simulink library "mbed_targets_stm_arch_max"  (R2015a)
settings: Solver=ode45  StartTime=0.0  StopTime=10.0  RelTol=1e-3
libraries: mbed_lib x5, mbed_targets_stm_disco_f407 x1
settings Model: CovSFcnEnable=off  Creator=oh  LastModifiedBy=Stuv
settings DebuggingCC: SolverPrmCheckMsg=warning

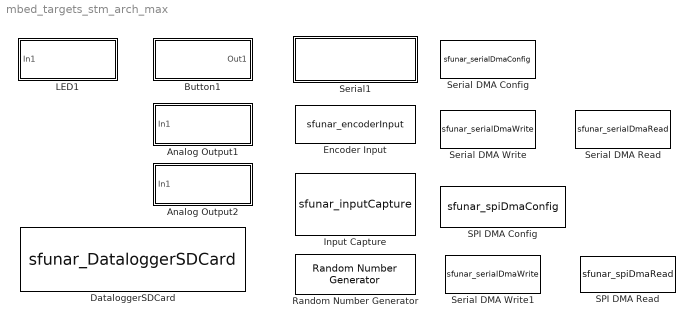
== system mbed_targets_stm_arch_max ==
  Analog Output1 : Subsystem  mask{Parameter1=0}
      mask Display:
      | offset=0.7;
      | plot([0+offset:0.025:0.25+offset],0.3*sin(2*pi*[0:0.1:1])+0.5)
      | port_label('input',1,['DAC1 (PA.4)']);
  Analog Output2 : Subsystem
      mask Display:
      | offset=0.7;
      | plot([0+offset:0.025:0.25+offset],0.3*sin(2*pi*[0:0.1:1])+0.5)
      | port_label('input',1,['DAC2 (PA.5)']);
  Button1 : Subsystem  mask{Parameter1=0}
      mask Display:
      | plot([0 0.15 0.15 0.35 0.35 0.5],[0.3 0.3 0.7 0.7 0.3 0.3])
      | port_label('output',1,['UsrBtn1']);
  DataloggerSDCard : S-Function  FunctionName=sfunar_DataloggerSDCard  Parameters=uint8(mosi_port), uint8(mosi_pin), uint8(miso_port), uint8(miso_pin), uint8(sclk_port), uint8(sclk_pin), uint8(cs_port), uint8(cs_pin), TypeInputPorts, SampleTime, uint8(errEn), uint32(BufferSize)  mask(Write csv style String into a file on SD Card){mosi_port=C, mosi_pin=3, miso_port=C, miso_pin=2, sclk_port=B, sclk_pin=10, cs_port=E, cs_pin=2, BufferSize=100, TypeInputPorts={ 'uint8' 8 'int8' 4 'bool' 1 }, TypeOfInputs={'8*uint8' '4*int8' '1*bool'}, errEn=on, SampleTime=-1}
      mask prompts: mosi_port "MOSI: Port"; mosi_pin "Pin"; miso_port "MISO: Port"; miso_pin "Pin"; sclk_port "SCLK: Port"; sclk_pin "Pin"; cs_port "CS: Port"; cs_pin "Pin"; BufferSize "Buffer Size"; TypeInputPorts "Type of Inputs"; TypeOfInputs "Type of Inputs"; errEn "Enable error output port"; SampleTime "Sample time (-1 for inherited):"
      mask help:
      | Parameters:
      | Serial Port:
      |  select Serial Port - corresponding config block is neccessary
      |
      | Type of Inputs:
      | List of 2-tuples
      |  1. item: Port width
      |  2. item: Port data type (single, double, int8, int16, int32, int64, uint8, uint16, uint32, uint64, bool)
      |  e.g.: {'8*uint8' '4*int8' '1*bool'}
      mask TypeOptions mosi_port: A | B | C | D | E | F
      mask TypeOptions mosi_pin: 0 | 1 | 2 | 3 | 4 | 5 | 6 | 7 | 8 | 9 | 10 | 11 | 12 | 13 | 14 | 15
      mask TypeOptions miso_port: A | B | C | D | E | F
      mask TypeOptions miso_pin: 0 | 1 | 2 | 3 | 4 | 5 | 6 | 7 | 8 | 9 | 10 | 11 | 12 | 13 | 14 | 15
      mask TypeOptions sclk_port: A | B | C | D | E | F
      mask TypeOptions sclk_pin: 0 | 1 | 2 | 3 | 4 | 5 | 6 | 7 | 8 | 9 | 10 | 11 | 12 | 13 | 14 | 15
      mask TypeOptions cs_port: A | B | C | D | E | F
      mask TypeOptions cs_pin: 0 | 1 | 2 | 3 | 4 | 5 | 6 | 7 | 8 | 9 | 10 | 11 | 12 | 13 | 14 | 15
      mask Callback TypeOfInputs:
      | cfg=eval(get_param(gcb,'TypeOfInputs'));
      | str={};
      | 
      | for i=1:size(cfg,2)
      |     res = strsplit(cfg{i}, '*');
      |     if isempty(str)
      |         str = strjoin({['''' res{2} ''''] res{1}});
      |     else
      |         str = strjoin({str ['''' res{2} ''''] res{1}});
      |     end
      | end
      | str = strjoin({'{' str '}'});
      | 
      | set_param(gcb,'TypeInputPorts', str);
      mask Display:
      | disp(['Datalogger SDCard\n\n']);
      | disp(['\n\nMOSI: P' mosi_port+64 '_' num2str(mosi_pin-1) ', MISO: P' miso_port+64, '_' num2str(miso_pin-1)  '\nSCLK: P' sclk_port+64, '_' num2str(sclk_pin-1)  ', CS: P' cs_port+64, '_' num2str(cs_pin-1)]);
      | for i=1:2:size(TypeInputPorts,2)
      |     port_label('input',(i+1)/2, [TypeInputPorts{i} ':' num2str(TypeInputPorts{i+1})]);
      | end
      | if errEn
      |     port_label('output',1,'Error');
      | end
  Encoder Input : S-Function  FunctionName=sfunar_encoderInput  Parameters=SampleTime, uint8(TimerNumber), uint8(EncoderMode), uint8(Ti1Port), uint8(Ti1Pin), uint8(Ti2Port), uint8(Ti2Pin), uint8(InputMode), uint16(Resolution)  mask{TimerNumber=TIM1, EncoderMode=TI1, Ti1Port=A, Ti1Pin=0, Ti2Port=A, Ti2Pin=0, InputMode=PullNone, Resolution=65535, SampleTime=-1}
      mask prompts: TimerNumber "Timer number:"; EncoderMode "Encoder Mode:"; Ti1Port "TI1 Port"; Ti1Pin "TI1 Pin"; Ti2Port "TI2 Port"; Ti2Pin "TI2 Pin"; InputMode "Input Mode (GPIO):"; Resolution "Resolution (Pulses/Rev):"; SampleTime "Sample time: (-1 for inherited)"
      mask TypeOptions TimerNumber: TIM1 | TIM2 | TIM3 | TIM4 | TIM5 | TIM8
      mask TypeOptions EncoderMode: TI1 | TI2 | TI1 and TI2
      mask TypeOptions Ti1Port: A | B | C | D | E | F
      mask TypeOptions Ti1Pin: 0 | 1 | 2 | 3 | 4 | 5 | 6 | 7 | 8 | 9 | 10 | 11 | 12 | 13 | 14 | 15
      mask TypeOptions Ti2Port: A | B | C | D | E | F
      mask TypeOptions Ti2Pin: 0 | 1 | 2 | 3 | 4 | 5 | 6 | 7 | 8 | 9 | 10 | 11 | 12 | 13 | 14 | 15
      mask TypeOptions InputMode: PullNone | PullUp | PullDown
      mask DialogControl DescTextVar Prompt: Hardware Encoder für STM32F4xx
      mask Display:
      | port_label('input',1,'Reset');
      | disp(['Timer ' num2str(TimerNumber) '\n\n']);
      | disp(['\nTI1:P' Ti1Port+64 '.' num2str(Ti1Pin-1) '\n' 'TI2:P' Ti2Port+64 '.' num2str(Ti2Pin-1) ]);
      | port_label('output',1,'Angle');
      | port_label('output',2,'RAW');
  Input Capture : S-Function  FunctionName=sfunar_inputCapture  Parameters=SampleTime, TimerNumber, Frequency, Ti1Active, Ti1Port, Ti1Pin, Ti1Pupd, Ti2Active, Ti2Port, Ti2Pin, Ti2Pupd, Ti3Active, Ti3Port, Ti3Pin, Ti3Pupd, Ti4Active, Ti4Port, Ti4Pin, Ti4Pupd, OutputMode  mask{TimerNumber=1, Frequency=1000000, OutputMode=Raw, Ti1Active=Rising, Ti1Port=A, Ti1Pin=0, Ti1Pupd=PullNone, Ti2Active=None, Ti2Port=A, Ti2Pin=0, Ti2Pupd=PullNone, Ti3Active=None, Ti3Port=A, Ti3Pin=0, Ti3Pupd=PullNone, Ti4Active=None, Ti4Port=A, Ti4Pin=0, Ti4Pupd=PullNone, SampleTime=-1}
      mask prompts: TimerNumber "Timer"; OutputMode "Output mode"; Ti1Active "Activate TI1"; Ti1Port "TI1 Port"; Ti1Pin "TI1 Pin"; Ti1Pupd "TI1 Pull type"; Ti2Active "Activate TI2"; Ti2Port "TI2 Port"; Ti2Pin "TI2 Pin"; Ti2Pupd "Ti2 Pull type"; Ti3Active "Activate TI3"; Ti3Port "TI3 Port"; Ti3Pin "TI3 Pin"; Ti3Pupd "TI3 Pull type"; Ti4Active "Activate TI4"; Ti4Port "TI4 Port"; Ti4Pin "TI4 Pin"; Ti4Pupd "TI4 Pull type"; SampleTime "Sample time (-1 for inherited):"
      mask TypeOptions TimerNumber: 1 | 2 | 3 | 4 | 5 | 8 | 9 | 10 | 11 | 12 | 13 | 14 | 15 | 16 | 17 | 20
      mask TypeOptions OutputMode: Raw | Period | Frequency
      mask TypeOptions Ti1Active: None | Rising | Falling | Both
      mask TypeOptions Ti1Port: A | B | C | D | E | F
      mask TypeOptions Ti1Pin: 0 | 1 | 2 | 3 | 4 | 5 | 6 | 7 | 8 | 9 | 10 | 11 | 12 | 13 | 14 | 15
      mask TypeOptions Ti1Pupd: PullNone | PullUp | PullDown
      mask TypeOptions Ti2Active: None | Rising | Falling | Both
      mask TypeOptions Ti2Port: A | B | C | D | E | F
      mask TypeOptions Ti2Pin: 0 | 1 | 2 | 3 | 4 | 5 | 6 | 7 | 8 | 9 | 10 | 11 | 12 | 13 | 14 | 15
      mask TypeOptions Ti2Pupd: PullNone | PullUp | PullDown
      mask TypeOptions Ti3Active: None | Rising | Falling | Both
      mask TypeOptions Ti3Port: A | B | C | D | E | F
      mask TypeOptions Ti3Pin: 0 | 1 | 2 | 3 | 4 | 5 | 6 | 7 | 8 | 9 | 10 | 11 | 12 | 13 | 14 | 15
      mask TypeOptions Ti3Pupd: PullNone | PullUp | PullDown
      mask TypeOptions Ti4Active: None | Rising | Falling | Both
      mask TypeOptions Ti4Port: A | B | C | D | E | F
      mask TypeOptions Ti4Pin: 0 | 1 | 2 | 3 | 4 | 5 | 6 | 7 | 8 | 9 | 10 | 11 | 12 | 13 | 14 | 15
      mask TypeOptions Ti4Pupd: PullNone | PullUp | PullDown
      mask Display:
      | disp(['Timer ' num2str(TimerNumber) '\n']);
      | disp('\n Input Capture');
      | port = 1;
      | 
      | if Ti1Active > 1
      |     port_label('output',port,['P' Ti1Port+64 '.' num2str(Ti1Pin-1)]);
      |     port = port + 1;
      | end
      | 
      | if Ti2Active > 1
      |     port_label('output',port,['P' Ti2Port+64 '.' num2str(Ti2Pin-1)]);
      |     port = port + 1;
      | end
      | 
      | if Ti3Active > 1
      |     port_label('output',port,['P' Ti3Port+64 '.' num2str(Ti3Pin-1)]);
      |     port = port + 1;
      | end
      | 
      | if Ti4Active > 1
      |     port_label('output',port,['P' Ti4Port+64 '.' num2str(Ti4Pin-1)]);
      |     port = port + 1;
      | end
  LED1 : Subsystem  mask{Parameter1=0}
      mask Display:
      | plot([0.5 0.65 0.65 0.85 0.85 1],[0.3 0.3 0.7 0.7 0.3 0.3])
      | port_label('input',1,['LED1']);
  Random Number Generator : mbed_targets_stm_disco_f407/Random Number Generator  SampleTime=-1
  SPI DMA Config : S-Function  FunctionName=sfunar_spiDmaConfig  Parameters=uint8(SpiPort), uint8(MosiPort), uint8(MosiPin), uint8(MisoPort), uint8(MisoPin), uint8(SclkPort), uint8(SclkPin), uint8(NssPort), uint8(NssPin), uint8(SlaveFlag), uint8(Frequency)  mask{SpiPort=SPI 1, MosiPort=A, MosiPin=0, MisoPort=A, MisoPin=0, SclkPort=A, SclkPin=0, NssPort=A, NssPin=0, SlaveFlag=off, Frequency=2}
      mask prompts: SpiPort "SPI Port"; MosiPort "MOSI Port"; MosiPin "MOSI Pin"; MisoPort "MISO Port"; MisoPin "MISO Pin"; SclkPort "SCLK Port"; SclkPin "SCLK Pin"; NssPort "NSS Port"; NssPin "NSS Pin"; SlaveFlag "SPI Slave"; Frequency "Baud rate prescaler"
      mask TypeOptions SpiPort: SPI 1 | SPI 2 | SPI 3 | SPI 4 | SPI 5
      mask TypeOptions MosiPort: A | B | C | D | E | F
      mask TypeOptions MosiPin: 0 | 1 | 2 | 3 | 4 | 5 | 6 | 7 | 8 | 9 | 10 | 11 | 12 | 13 | 14 | 15
      mask TypeOptions MisoPort: A | B | C | D | E | F
      mask TypeOptions MisoPin: 0 | 1 | 2 | 3 | 4 | 5 | 6 | 7 | 8 | 9 | 10 | 11 | 12 | 13 | 14 | 15
      mask TypeOptions SclkPort: A | B | C | D | E | F
      mask TypeOptions SclkPin: 0 | 1 | 2 | 3 | 4 | 5 | 6 | 7 | 8 | 9 | 10 | 11 | 12 | 13 | 14 | 15
      mask TypeOptions NssPort: A | B | C | D | E | F
      mask TypeOptions NssPin: 0 | 1 | 2 | 3 | 4 | 5 | 6 | 7 | 8 | 9 | 10 | 11 | 12 | 13 | 14 | 15
      mask TypeOptions Frequency: 2 | 4 | 8 | 16 | 32 | 64 | 128 | 256
      mask Display:
      | if SlaveFlag == 1
      | disp(['SPI ' num2str(SpiPort) ' Slave DMA\n\n']);
      | else
      | disp(['SPI ' num2str(SpiPort) ' Master DMA\n\n']);
      | end
      | 
      | disp(['MOSI:P' MosiPort+64 '.' num2str(MosiPin-1) ', MISO:P' MisoPort+64 '.' num2str(MisoPin-1)]);
      | 
      | disp(['\n\nSCLK:P' SclkPort+64 '.' num2str(SclkPin-1) ', NSS:P' NssPort+64 '.' num2str(NssPin-1)]);
  SPI DMA Read : S-Function  FunctionName=sfunar_spiDmaRead  Parameters=SampleTime, uint8(SpiPort), uint32(RxBuffer), uint32(PortWidth)  mask{SpiPort=1, RxBuffer=10, PortWidth=5, SampleTime=-1}
      mask prompts: SpiPort "SPI Port:"; RxBuffer "DMA buffer size:"; PortWidth "specify data port width:"; SampleTime "Sample time (-1 for inherited):"
      mask TypeOptions SpiPort: 1 | 2 | 3 | 4 | 5
      mask Display:
      | disp(['SPI' num2str(SpiPort) ' DMA Read']);
      | 
      | port_label('output',1,'d');
      | 
      | port_label('output',2,'n')
  Serial DMA Config : S-Function  FunctionName=sfunar_serialDmaConfig  Parameters=SerialPort, TxPort, TxPin, RxPort, RxPin, uint32(BaudRate)  mask{SerialPort=1, TxPort=A, TxPin=0, RxPort=A, RxPin=0, BaudRate=115200}
      mask prompts: SerialPort "Serial Port:"; TxPort "Port Name (TX):"; TxPin "Pin Number (0-15)"; RxPort "Port Name (RX):"; RxPin "Pin Name (0-15)"; BaudRate "Baud Rate:"
      mask TypeOptions SerialPort: 1 | 2 | 3 | 4 | 5 | 6
      mask TypeOptions TxPort: A | B | C | D | E | F
      mask TypeOptions TxPin: 0 | 1 | 2 | 3 | 4 | 5 | 6 | 7 | 8 | 9 | 10 | 11 | 12 | 13 | 14 | 15
      mask TypeOptions RxPort: A | B | C | D | E | F
      mask TypeOptions RxPin: 0 | 1 | 2 | 3 | 4 | 5 | 6 | 7 | 8 | 9 | 10 | 11 | 12 | 13 | 14 | 15
      mask Display:
      | disp(['\nSerial ' num2str(SerialPort) ' DMA\n\n']);
      | disp(['\nTX:' TxPort+64 '.' num2str(TxPin-1) ', RX:' RxPort+64, '.' num2str(RxPin-1)]);
  Serial DMA Read : S-Function  FunctionName=sfunar_serialDmaRead  Parameters=SampleTime, SerialPort, uint32(RxBuffer), int32(PortWidth)  mask{SerialPort=1, RxBuffer=10, PortWidth=5, SampleTime=-1}
      mask prompts: SerialPort "Serial Port:"; RxBuffer "DMA buffer size:"; PortWidth "specify data port width:"; SampleTime "Sample time (-1 for inherited):"
      mask TypeOptions SerialPort: 1 | 2 | 3 | 4 | 5 | 6
      mask Display:
      | disp(['Serial' num2str(SerialPort) ' DMA Read']);
      | port_label('output',1,'d');
      | port_label('output',2,'n');
  Serial DMA Write : S-Function  FunctionName=sfunar_serialDmaWrite  Parameters=SampleTime, SerialPort  mask{SerialPort=1, SampleTime=-1}
      mask prompts: SerialPort "Serial Port:"; SampleTime "Sample time (-1 for inherited):"
      mask TypeOptions SerialPort: 1 | 2 | 3 | 4 | 5 | 6
      mask Display: disp(['Serial' num2str(SerialPort) ' DMA Write']);
  Serial DMA Write1 : S-Function  FunctionName=sfunar_serialDmaWrite  Parameters=SampleTime, SerialPort, numData  mask{SerialPort=1, numData=off, SampleTime=-1}
      mask prompts: SerialPort "Serial Port:"; numData "Enable Number of Data Port"; SampleTime "Sample time (-1 for inherited):"
      mask TypeOptions SerialPort: 1 | 2 | 3 | 4 | 5 | 6
      mask Display: disp(['Serial' num2str(SerialPort) ' DMA Write']);
  Serial1 : Subsystem  mask{Parameter1=0}
      mask Display: disp(['Serial1(USB)\nTX:PC_6, RX:PC_7'])

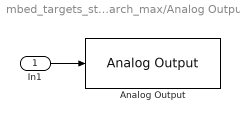
== system mbed_targets_stm_arch_max/Analog Output1 ==
  In1 : Inport
  Analog Output : mbed_lib/GPIO/Analog Output  SParameter2=A  SParameter1=4  inputVariant=Double: 0 - 1.0f  SampleTime=-1
  wires:
  In1/1 -> Analog Output/1

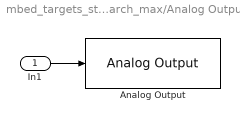
== system mbed_targets_stm_arch_max/Analog Output2 ==
  In1 : Inport
  Analog Output : mbed_lib/GPIO/Analog Output  SParameter2=A  SParameter1=5  inputVariant=Double: 0 - 1.0f  SampleTime=-1
  wires:
  In1/1 -> Analog Output/1

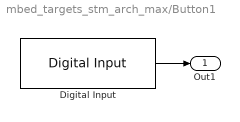
== system mbed_targets_stm_arch_max/Button1 ==
  Digital Input : mbed_lib/GPIO/Digital Input  SParameter2=A  SParameter1=0  SParameter3=PullDefault  SampleTime=-1
  Out1 : Outport
  wires:
  Digital Input/1 -> Out1/1

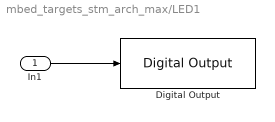
== system mbed_targets_stm_arch_max/LED1 ==
  In1 : Inport
  Digital Output : mbed_lib/GPIO/Digital Output  SParameter2=B  SParameter1=3  SParameter3=PullDefault  SampleTime=-1
  wires:
  In1/1 -> Digital Output/1

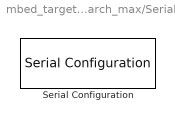
== system mbed_targets_stm_arch_max/Serial1 ==
  Serial Configuration : mbed_lib/Serial/Serial Configuration  SerialPort=1  TXPort=C  TXPin=6  RXPort=C  RXPin=7  BaudRate=9600
